simulink model "ROBOT_model"  (R2016b)
settings: Solver=ode5  StartTime=0.0  StopTime=10.0  FixedStep=0.01  RelTol=1e-3
libraries: simulink_need_slupdate x3
settings Model: Creator=davide  LastModifiedBy=davide

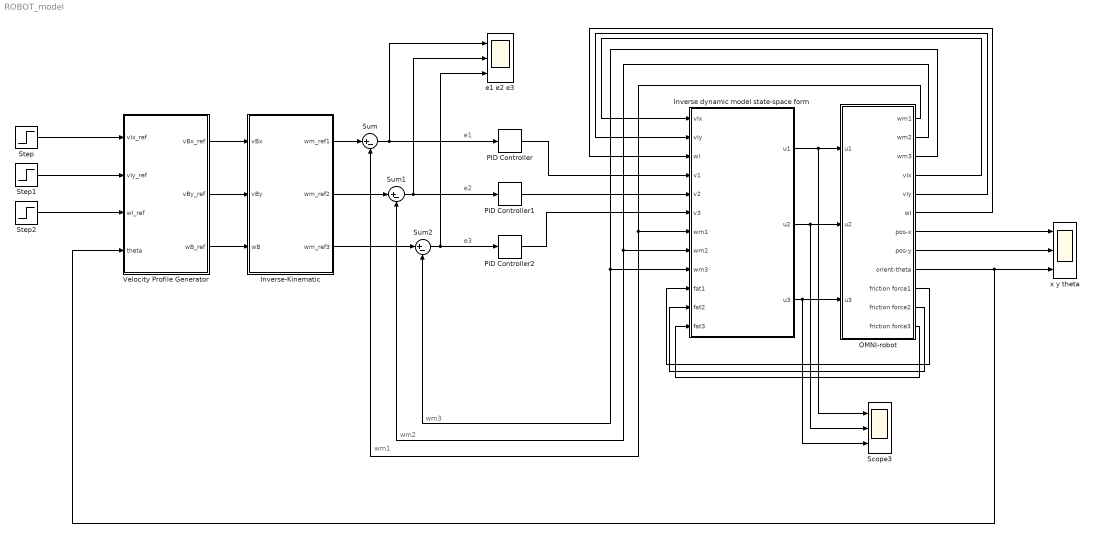
== system ROBOT_model ==
  note: wm3
  note: wm2
  note: wm1
  note: e3
  note: e2
  note: e1
  Inverse dynamic model state-space form : MATLAB Function  TreatAsAtomicUnit=on
  Inverse-Kinematic : MATLAB Function  TreatAsAtomicUnit=on
  OMNI-robot : Subsystem
  PID Controller : simulink_need_slupdate/PID Controller  P=40  I=571.43  D=0
  PID Controller1 : simulink_need_slupdate/PID Controller  P=40  I=571.43  D=0
  PID Controller2 : simulink_need_slupdate/PID Controller  P=40  I=571.43  D=0
  Scope3 : Scope  NumInputPorts=3
  Step : Step  SampleTime=0
  Step1 : Step  After=0  SampleTime=0
  Step2 : Step  After=0  SampleTime=0
  Sum : Sum  Inputs=|+-
  Sum1 : Sum  Inputs=|+-
  Sum2 : Sum  Inputs=|+-
  Velocity Profile Generator : MATLAB Function  TreatAsAtomicUnit=on
  e1 e2 e3 : Scope  NumInputPorts=3
  x y theta : Scope  NumInputPorts=3
  wires:
  Inverse dynamic model state-space form/1(u1) -> Scope3/1, OMNI-robot/1(u1)
  Inverse dynamic model state-space form/2(u2) -> Scope3/2, OMNI-robot/2(u2)
  Inverse dynamic model state-space form/3(u3) -> Scope3/3, OMNI-robot/3(u3)
  OMNI-robot/2(wm2) -> Sum1/2, Inverse dynamic model state-space form/8(wm2)
  OMNI-robot/3(wm3) -> Sum2/2, Inverse dynamic model state-space form/9(wm3)
  OMNI-robot/10(friction force1) -> Inverse dynamic model state-space form/10(fat1)
  OMNI-robot/11(friction force2) -> Inverse dynamic model state-space form/11(fat2)
  OMNI-robot/12(friction force3) -> Inverse dynamic model state-space form/12(fat3)
  OMNI-robot/4(vIx) -> Inverse dynamic model state-space form/1(vIx)
  OMNI-robot/5(vIy) -> Inverse dynamic model state-space form/2(vIy)
  OMNI-robot/6(wI) -> Inverse dynamic model state-space form/3(wI)
  PID Controller1/1 -> Inverse dynamic model state-space form/5(v2)
  PID Controller/1 -> Inverse dynamic model state-space form/4(v1)
  PID Controller2/1 -> Inverse dynamic model state-space form/6(v3)
  OMNI-robot/8(pos-y) -> x y theta/2
  OMNI-robot/7(pos-x) -> x y theta/1
  Sum2/1 -> e1 e2 e3/3, PID Controller2/1
  Sum1/1 -> e1 e2 e3/2, PID Controller1/1
  Inverse-Kinematic/1(wm_ref1) -> Sum/1
  Inverse-Kinematic/2(wm_ref2) -> Sum1/1
  Inverse-Kinematic/3(wm_ref3) -> Sum2/1
  Sum/1 -> e1 e2 e3/1, PID Controller/1
  OMNI-robot/1(wm1) -> Sum/2, Inverse dynamic model state-space form/7(wm1)
  Velocity Profile Generator/1(vBx_ref) -> Inverse-Kinematic/1(vBx)
  Velocity Profile Generator/2(vBy_ref) -> Inverse-Kinematic/2(vBy)
  Velocity Profile Generator/3(wB_ref) -> Inverse-Kinematic/3(wB)
  Step/1 -> Velocity Profile Generator/1(vIx_ref)
  Step2/1 -> Velocity Profile Generator/3(wI_ref)
  Step1/1 -> Velocity Profile Generator/2(vIy_ref)
  OMNI-robot/9(orient-theta) -> Velocity Profile Generator/4(theta), x y theta/3

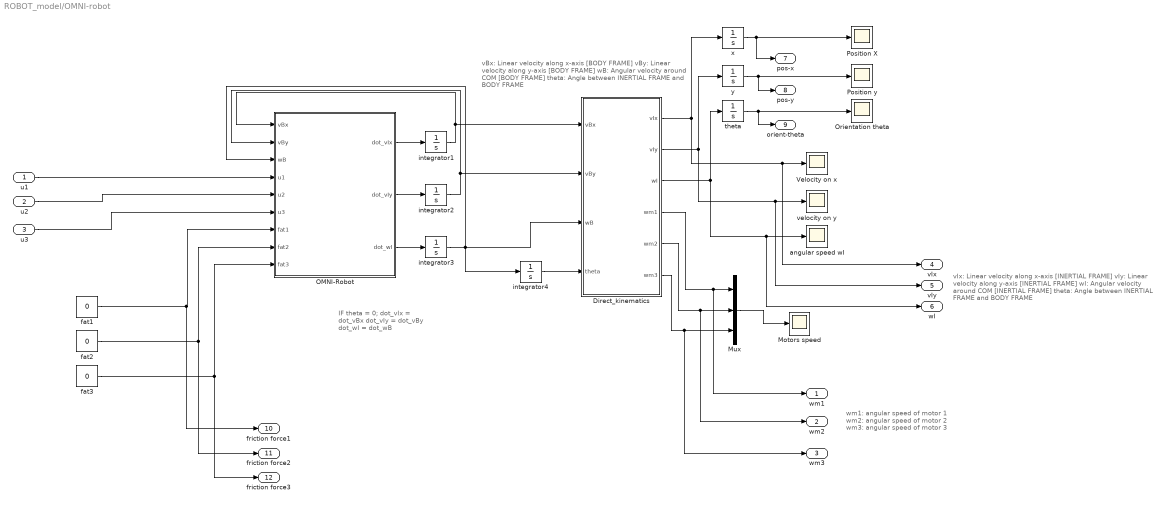
== system ROBOT_model/OMNI-robot ==
  note: wm1: angular speed of motor 1
      | wm2: angular speed of motor 2
      | wm3: angular speed of motor 3
  note: vIx: Linear velocity along x-axis   [INERTIAL FRAME]
      | vIy: Linear velocity along y-axis   [INERTIAL FRAME]
      | wI: Angular velocity around COM [INERTIAL FRAME]
      | theta: Angle between INERTIAL FRAME and BODY FRAME
  note: vBx: Linear velocity along x-axis   [BODY FRAME]
      | vBy: Linear velocity along y-axis   [BODY FRAME]
      | wB: Angular velocity around COM [BODY FRAME]
      | theta: Angle between INERTIAL FRAME and BODY FRAME
  note: IF theta = 0;
      |
      | dot_vIx = dot_vBx
      | dot_vIy = dot_vBy
      | dot_wI  = dot_wB
  u1 : Inport
  u2 : Inport  Port=2
  u3 : Inport  Port=3
  Direct_kinematics : MATLAB Function  TreatAsAtomicUnit=on
  Motors speed : Scope
  Mux : Mux  Inputs=3
  OMNI-Robot : MATLAB Function  TreatAsAtomicUnit=on
  Orientation theta : Scope
  Position X : Scope
  Position y : Scope
  Velocity on x : Scope
  angular speed wI : Scope
  fat1 : Constant  Value=0
  fat2 : Constant  Value=0
  fat3 : Constant  Value=0
  integrator{1..4} (4 alike) : Integrator
  theta : Integrator
  velocity on y : Scope
  x : Integrator
  y : Integrator
  wm1 : Outport
  wm2 : Outport  Port=2
  wm3 : Outport  Port=3
  vIx : Outport  Port=4
  vIy : Outport  Port=5
  wI : Outport  Port=6
  pos-x : Outport  Port=7
  pos-y : Outport  Port=8
  orient-theta : Outport  Port=9
  friction force1 : Outport  Port=10
  friction force2 : Outport  Port=11
  friction force3 : Outport  Port=12
  wires:
  OMNI-Robot/2(dot_vIy) -> integrator2/1
  OMNI-Robot/3(dot_wI) -> integrator3/1
  Direct_kinematics/4(wm1) -> wm1/1, Mux/1
  Direct_kinematics/5(wm2) -> wm2/1, Mux/2
  OMNI-Robot/1(dot_vIx) -> integrator1/1
  integrator1/1 -> Direct_kinematics/1(vBx), OMNI-Robot/1(vBx)
  integrator2/1 -> Direct_kinematics/2(vBy), OMNI-Robot/2(vBy)
  integrator4/1 -> Direct_kinematics/4(theta)
  integrator3/1 -> OMNI-Robot/3(wB), Direct_kinematics/3(wB), integrator4/1
  Direct_kinematics/2(vIy) -> vIy/1, velocity on y/1, y/1
  Direct_kinematics/3(wI) -> wI/1, angular speed wI/1, theta/1
  theta/1 -> orient-theta/1, Orientation theta/1
  y/1 -> pos-y/1, Position y/1
  x/1 -> Position X/1, pos-x/1
  Direct_kinematics/1(vIx) -> vIx/1, Velocity on x/1, x/1
  Direct_kinematics/6(wm3) -> wm3/1, Mux/3
  Mux/1 -> Motors speed/1
  fat1/1 -> friction force1/1, OMNI-Robot/7(fat1)
  fat2/1 -> friction force2/1, OMNI-Robot/8(fat2)
  fat3/1 -> friction force3/1, OMNI-Robot/9(fat3)
  u1/1 -> OMNI-Robot/4(u1)
  u2/1 -> OMNI-Robot/5(u2)
  u3/1 -> OMNI-Robot/6(u3)

== matlab function ROBOT_model/OMNI-robot/Direct_kinematics ==
  data: vBx input; vIx output; vBy input; wB input; theta input; vIy output; wI output; wm1 output; wm2 output; wm3 output

function [vIx,vIy,wI,wm1,wm2,wm3] = Direct_KIN(vBx,vBy,wB,theta)

%%%%% INPUTS %%%%%
% vBx    =  Linear acceleration along x-axis    [BODY-FRAME]
% vBy    =  Linear acceleration along y-axis    [BODY-FRAME]
%  wB    =  Angular acceleration around z-axis  [BODY-FRAME]
% theta  =  angle between Inertial frame and Body frame 

%%%%% OUTPUTS %%%%
% vIx     =   linear velocity along x-direction  [INERTIAL-FRAME]
% vIy     =   linear velocity along x-direction  [INERTIAL-FRAME]
% wI      =   Angular velocity around z-axis     [INERTIAL-FRAME]
% Wm1     =   Angular speed of motor 1
% Wm2     =   Angular speed of motor 2
% Wm3     =   Angular speed of motor 3


%%%% STRUCTURAL PARAMETERS %%%%
N=19; % Reduction Ratio of the motors (adimensional)
eta=0.83; % Mechanical coupling efficiency (adimensional)
l=0.09;  % Distance between base center and wheel center [m]
rw=0.072; % Wheel radius [m]

%%%% GEOMETRICAL PARAMETERS %%%%
B = [0 cos(pi/6) -cos(pi/6); -1 sin(pi/6) sin(pi/6); l l l]; % Geometrical Jacobian with pi/6 = 30° = delta (4.6)
Tr = [cos(theta) -sin(theta) 0; sin(theta) cos(theta) 0; 0 0 1]; % Rotation Matrix (4.2)
Tri = inv(Tr);
%% TRANSFORMATION FROM BODY-FRAME TO INERTIAL-FRAME COORDINATES
% We now implement the direct kinematic model of the OMNI-robot as follows (4.10):

T=Tri*[vBx;vBy;wB]; 

% the obtained vector T is the vector of linear and angular velocities in
% INERTIAL FRAME and its components are defined as follows:
vIx=T(1,:);% linear velocity along x-direction  [INERTIAL-FRAME]
vIy=T(2,:);% linear velocity along y-direction  [INERTIAL-FRAME]
wI=T(3,:); % Angular velocity around z-axis     [INERTIAL-FRAME]
% END

%% INVERSE KINEMATIC - COMPUTE THE MOTORS ANGULAR SPEEDS 
% We now implement the inverse kinematic model of the OMNI-robot as
% follows (4.11):

W=((eta*N)/rw)*B'*[vBx;vBy;wB];

% the obtained vector W is the vector of motors angular speed and its 
% components are defined as follows:
wm1=W(1,:); % Angular speed of motor 1
wm2=W(2,:); % Angular speed of motor 2
wm3=W(3,:); % Angular speed of motor 3
% END

== matlab function ROBOT_model/OMNI-robot/OMNI-Robot ==
  data: vBx input; dot_vIx output; vBy input; wB input; u1 input; u2 input; u3 input; fat1 input; fat2 input; fat3 input; dot_vIy output; dot_wI output
function [dot_vIx,dot_vIy,dot_wI] = Robot_model(vBx,vBy,wB,u1,u2,u3,fat1,fat2,fat3)

% fat1, fat2, and fat3 are the friction forces, for now we will consider an
% ideal case with NO FRICTIONS.

%%%%% INPUTS %%%%%
% vBx    =   linear velocity along x-direction  [BODY-FRAME]
% vBy    =   linear velocity along y-direction  [BODY-FRAME]
% wB     =   angular velocity around COM        [BODY-FRAME]
% u1    =   real rotational speed of the wheel 1
% u2    =   real rotational speed of the wheel 2
% u3    =   real rotational speed of the wheel 3
% fat1  =   friction force on wheel 1
% fat2  =   friction force on wheel 2
% fat3  =   friction force on wheel 3

%%%% OUTPUTS %%%%
% dot_vIx    =  Linear acceleration along x-axis    [INERTIAL-FRAME]
% dot_vIy    =  Linear acceleration along y-axis    [INERTIAL-FRAME]
% dot_wI     =  Angular acceleration around z-axis  [INERTIAL-FRAME]

%%%% STRUCTURAL PARAMETERS %%%%
N=19; % Reduction Ratio of the motors (adimensional)
eta=0.83; % Mechanical coupling efficiency (adimensional)
kt=0.0059; % Torque constant [Nm/A]
kem=0.0059;  % EMF constanht [Vs/rad]
Jm=3.88e-7; % Motor Inertia [kgm^2]
J=2.125; % Inertia of mobile base [kgm^2]
l=0.09;  % Distance between base center and wheel center [m]
rw=0.072; % Wheel radius [m]
M=1.830; % Mass of the mobile base [Kg]
R=1.710; % Motor resistance [Ohm]
bo = 2.4e-6; % Damping constant for motor load coupling

% PARAMETER INITIALIZATION
dot_vIx=0;
dot_vIy=0;
dot_wI=0;
% END

%%%% GEOMETRICAL PARAMETERS %%%%
H = [1/M 0 0; 0 1/M 0; 0 0 1/J]; % inverse of the mass matrix (4.20)
B = [0 cos(pi/6) -cos(pi/6); -1 sin(pi/6) sin(pi/6); l l l]; % Geometrical Jacobian with pi/6 = 30° = delta (4.6)
I = [1 0 0; 0 1 0; 0 0 1]; % Identity matrix
G = I+(H*B*B.'*((((eta*N)^2)*Jm)/(rw^2)));  % factorization for dynamic equation re-writing --> see pag.41 Thiago Thesis
Gi=inv(G);


%%%%%%% DYNAMIC MODEL IMPLEMENTATION %%%%%%%

% We now implement the dynamic model of the Omnidirectional-Robot obtained
% by the geometrical analysis of the structure plus the wheel-motor dynamic
% system (3 sets of wheel-motor)  (4.33)

A= (-(Gi*H*B*B.'*(((kt*kem)/R)+bo).*(((eta*N)^2)/(rw^2))*[vBx;vBy;wB])+Gi*H*B*((kt*eta*N)/(rw*R))*[u1;u2;u3])-Gi*H*B*[fat1;fat2;fat3];

% A is the obtained vector of the accelerations [INERTIAL FRAME] with each
% of its components defined as follows:
dot_vIx=A(1,:);  % acceleration along x-axis       [INERTIAL FRAME]
dot_vIy=A(2,:);  % acceleration along y-axis       [INERTIAL FRAME]
dot_wI=A(3,:);   % angular acceleration around COM [INERTIAL FRAME]

%% PLEASE REMEMBER THE FUNDAMENTAL RELATIONSHIP:
% if we assume for simplicity that we want to keep constant the orientation
% of the robot during its displacement along its trajectory we can assume
% theta=0° and due to this simplification we have dot_theta=0 (theta is the
% angle between Inertial frame and Body frame). With this result we can
% write :
%  dot_vIx = dot_vBx
%  dot_vIy = dot_vBx
%  dot_wI  = dot_wB

== matlab function ROBOT_model/Inverse dynamic model state-space form ==
  data: vIx input; vIy input; wI input; u1 output; v1 input; v2 input; v3 input; wm1 input; wm2 input; wm3 input; fat1 input; fat2 input; fat3 input; u2 output; u3 output
function [u1,u2,u3] = Linearization(vIx,vIy,wI,v1,v2,v3,wm1,wm2,wm3,fat1,fat2,fat3)

% fat1, fat2, and fat3 are the friction forces, for now we will consider an
% ideal case with NO FRICTIONS.

N=19; % Reduction Ratio of the motors (adimensional)
eta=0.83; % Mechanical coupling efficiency (adimensional)
kt=0.0059; % Torque constant [Nm/A]
kem=0.0059;  % EMF constanht [Vs/rad]
Jm=3.88e-7; % Motor Inertia [kgm^2]
J=2.125; % Inertia of mobile base [kgm^2]
l=0.09;  % % Distance between base center and wheel center [m]
rw=0.07; % Radius of wheels [m]
M=1.830; % Mass of the mobile base [Kg]
R=1.710; % Motor resistance [Ohm]
bo = 2.4e-6; % Coupling Damping coefficient

% PARAMETERS INITIALIZATION
dot_vIx=0;
dot_vIy=0;
dot_wI=0;
% END

%%%% GEOMETRICAL PARAMETERS %%%%
H = [1/M 0 0; 0 1/M 0; 0 0 1/J]; % inverse of the mass matrix (4.20)
B = [0 cos(pi/6) -cos(pi/6); -1 sin(pi/6) sin(pi/6); l l l]; % Geometrical Jacobian with pi/6 = 30° = delta (4.6)
I = [1 0 0; 0 1 0; 0 0 1];
G = I+(H*B*B.'*((((eta*N)^2)*Jm)/(rw^2))); % factorization for dynamic equation re-writing --> see pag.41 Thiago Thesis

%% Inverse dynamic model in state-space form:
%    | x^{n} = f(x)+G(x)u
%    | y = x^{n}
%%%%%%%%%%%%%%%%%%%%%%%%%%%%%%%%%%%%%%%%%%%%%%%%%%%%%%%%%%%%%%%%%%%%%%%%%%%%%%%%
% TRANSITION MATRIX f(x)
%  f(x)=-Ai*Gi*H*B*(([fat1;fat2;fat3])+((kt*kem/R)+bo)*((eta*N)/rw)*[w1;w2;w3]))
% INPUT-MATRIX G(x)
%  G(x)=(Ai*Gi*H*B)*((kt*eta*N)/(R*rw));      
% STATE VECTOR x
%    x = [w1; w2; w3] (with w1,2,3 motors angular speeds)
% INPUT VECTOR u
%    u = [u1; u2; u3]
%%%%%%%%%%%%%%%%%%%%%%%%%%%%%%%%%%%%%%%%%%%%%%%%%%%%%%%%%%%%%%%%%%%%%%%%%%%%%%%%


Gi=inv(G);
Ai=((eta*N)/rw)*B.';  % factorization for dynamic equation re-writing --> see pag.41 Thiago Thesis (4.35)
Gx=(Ai*Gi*H*B)*((kt*eta*N)/(R*rw)); % INPUT-MATRIX G(x)
GxI=inv(Gx); % inverse of INPUT-MATRIX G(x)

%% INVERSE DYNAMIC MODEL IN STATE-SPACE FORM OF THE ROBOT
U=GxI*(Ai*Gi*H*B*[fat1;fat2;fat3]+(Ai*Gi*H*B*((kt*kem/R)+bo)*((eta*N)/rw)*[wm1;wm2;wm3]))+GxI*[v1;v2;v3];

% INPUT-VECTOR
u1=U(1,:);
u2=U(2,:);
u3=U(3,:);
% END

== matlab function ROBOT_model/Inverse-Kinematic ==
  data: vBx input; wm_ref1 output; vBy input; wB input; wm_ref2 output; wm_ref3 output
function [wm_ref1,wm_ref2,wm_ref3] = Inv_KIN(vBx,vBy,wB)

%%%%% INPUTS %%%%%
% vBx    =  Linear acceleration along x-axis    [BODY-FRAME]
% vBy    =  Linear acceleration along y-axis    [BODY-FRAME]
%  wB    =  Angular acceleration around z-axis  [BODY-FRAME]
%%%%% OUTPUTS %%%%
% Wm1     =   Angular speed of motor 1
% Wm2     =   Angular speed of motor 2
% Wm3     =   Angular speed of motor 3

%%%% STRUCTURAL PARAMETERS %%%%
N=19; % Reduction Ratio of the motors (adimensional)
eta=0.83; % Mechanical coupling efficiency (adimensional)
l=0.09;  % % Distance between base center and wheel center [m]
rw=0.07; % Radius of wheels [m]
B = [0 cos(pi/6) -cos(pi/6); -1 sin(pi/6) sin(pi/6); l l l]; % Geometrical Jacobian with pi/6 = 30° = delta (4.6)

%% INVERSE KINEMATIC - COMPUTE THE MOTORS ANGULAR SPEEDS 
% We now implement the inverse kinematic model of the OMNI-robot as
% follows (4.11):

% the obtained vector W is the vector of motors angular speed and its 
% components are defined as follows:
W=((eta*N)/rw)*B'*[vBx;vBy;wB];

wm_ref1=W(1,:); % Angular speed of motor 1 (reference value)
wm_ref2=W(2,:); % Angular speed of motor 2 (reference value)
wm_ref3=W(3,:); % Angular speed of motor 3 (reference value)
% END

== matlab function ROBOT_model/Velocity Profile Generator ==
  data: vIx_ref input; vBx_ref output; vIy_ref input; wI_ref input; vBy_ref output; wB_ref output; theta input
function [vBx_ref,vBy_ref,wB_ref] = Vel_prof(vIx_ref,vIy_ref,wI_ref,theta)
%%%%% INPUTS %%%%%
% vBx    =  Linear acceleration along x-axis    [BODY-FRAME]
% vBy    =  Linear acceleration along y-axis    [BODY-FRAME]
%  wB    =  Angular acceleration around z-axis  [BODY-FRAME]
% theta  =  angle between Inertial frame and Body frame 

%%%%% OUTPUTS %%%%
% vIx     =   linear velocity along x-direction  [INERTIAL-FRAME]
% vIy     =   linear velocity along x-direction  [INERTIAL-FRAME]
% wI      =   Angular velocity around z-axis     [INERTIAL-FRAME]
% Wm1     =   Angular speed of motor 1
% Wm2     =   Angular speed of motor 2
% Wm3     =   Angular speed of motor 3


%%%% STRUCTURAL PARAMETERS %%%%
N=19; % Reduction Ratio of the motors (adimensional)
eta=0.83; % Mechanical coupling efficiency (adimensional)
l=0.09;  % Distance between base center and wheel center [m]
rw=0.072; % Wheel radius [m]

%%%% GEOMETRICAL PARAMETERS %%%%
B = [0 cos(pi/6) -cos(pi/6); -1 sin(pi/6) sin(pi/6); l l l]; % Geometrical Jacobian with pi/6 = 30° = delta (4.6)

%% TRANSFORMATION FROM INERTIAL-FRAME COORDINATES TO BODY-FRAME COORDINATES
% We now implement the direct kinematic model of the OMNI-robot as follows (4.10):

T=[cos(theta) -sin(theta) 0; sin(theta) cos(theta) 0; 0 0 1]*[vIx_ref;vIy_ref;wI_ref]; 

% the obtained vector T is the vector of linear and angular velocities in
% INERTIAL FRAME and its components are defined as follows:
vBx_ref=T(1,:);% linear velocity along x-direction  [BODY-FRAME]
vBy_ref=T(2,:);% linear velocity along y-direction  [BODY-FRAME]
wB_ref=T(3,:); % Angular velocity around z-axis     [BODY-FRAME]
% END
